simulink library "limbo_algorithm_atomic_sub_chart_library"  (R2013b)
settings: Solver=ode45  StartTime=0.0  StopTime=10.0  RelTol=1e-3
libraries: legonxtlib x1
settings Model: Creator=mbiesiad  LastModifiedBy=grouleau

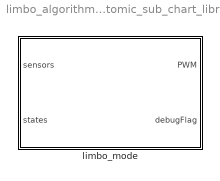
== system limbo_algorithm_atomic_sub_chart_library ==
  limbo_mode : Stateflow chart  TreatAsAtomicUnit=on

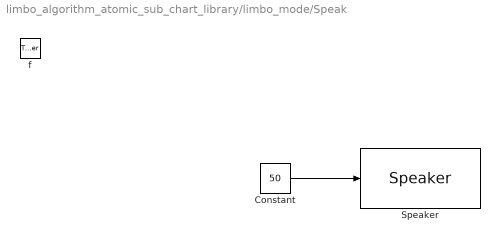
== system limbo_algorithm_atomic_sub_chart_library/limbo_mode/Speak ==
  f : TriggerPort  TriggerType=function-call
      settings: CopyFcn=Stateflow.SLINSF.SimulinkMan.removeBlockPreDeleteFcn  PreDeleteFcn=Stateflow.SLINSF.SimulinkMan.unsafePredeleteFcn
  Constant : Constant  Value=50
  Speaker : legonxtlib/Speaker  sinputMode=Volume only  sspeakerFreq=800  sspeakerVolume=50  sspeakerDuration=100
  wires:
  Constant/1 -> Speaker/1

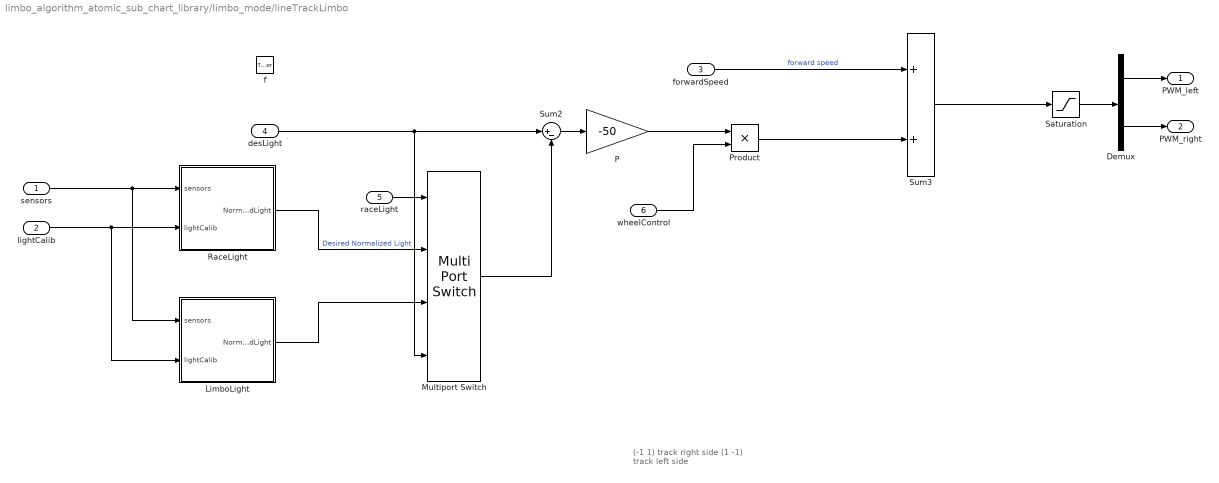
== system limbo_algorithm_atomic_sub_chart_library/limbo_mode/lineTrackLimbo ==
  note: (-1 1)  track right side
      | (1 -1)  track left side
  sensors : Inport  OutDataTypeStr=Bus: Sensors_Bus  PortDimensions=1  LockScale=on
  lightCalib : Inport  Port=2  OutDataTypeStr=Bus: Light_Bus  PortDimensions=1
  forwardSpeed : Inport  Port=3  OutDataTypeStr=single  PortDimensions=[1 2]
  desLight : Inport  Port=4  OutDataTypeStr=single  PortDimensions=1
  raceLight : Inport  Port=5  OutDataTypeStr=single  PortDimensions=1
  wheelControl : Inport  Port=6  OutDataTypeStr=single  PortDimensions=[1 2]
  f : TriggerPort  TriggerType=function-call
      settings: CopyFcn=Stateflow.SLINSF.SimulinkMan.removeBlockPreDeleteFcn  PreDeleteFcn=Stateflow.SLINSF.SimulinkMan.unsafePredeleteFcn
  Demux : Demux  Outputs=2
  LimboLight : Subsystem
  Multiport Switch : MultiPortSwitch
  P : Gain  Gain=-50
  Product : Product
  RaceLight : Subsystem
  Saturation : Saturate  UpperLimit=100  LowerLimit=-100  OutDataTypeStr=single
  Sum2 : Sum  Inputs=|+-
  Sum3 : Sum
  PWM_left : Outport  OutDataTypeStr=single  PortDimensions=1
  PWM_right : Outport  Port=2  OutDataTypeStr=single  PortDimensions=1
  wires:
  Saturation/1 -> Demux/1
  P/1 -> Product/1
  forwardSpeed/1 -> Sum3/1  "forward speed"
  Demux/2 -> PWM_right/1
  Demux/1 -> PWM_left/1
  Sum2/1 -> P/1
  desLight/1 -> Multiport Switch/4, Sum2/1  "Desired Normalized Light"
  sensors/1 -> LimboLight/1(sensors), RaceLight/1(sensors)
  lightCalib/1 -> LimboLight/2(lightCalib), RaceLight/2(lightCalib)
  LimboLight/1(NormalizedLight) -> Multiport Switch/3
  raceLight/1 -> Multiport Switch/1
  RaceLight/1(NormalizedLight) -> Multiport Switch/2
  Multiport Switch/1 -> Sum2/2
  wheelControl/1 -> Product/2
  Sum3/1 -> Saturation/1
  Product/1 -> Sum3/2

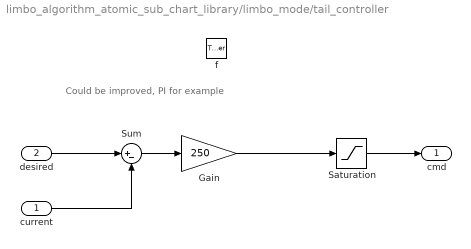
== system limbo_algorithm_atomic_sub_chart_library/limbo_mode/tail_controller ==
  note: Could be improved, PI for example
  current : Inport  OutDataTypeStr=single  PortDimensions=1
  desired : Inport  Port=2  OutDataTypeStr=single  PortDimensions=1
  f : TriggerPort  TriggerType=function-call
      settings: CopyFcn=Stateflow.SLINSF.SimulinkMan.removeBlockPreDeleteFcn  PreDeleteFcn=Stateflow.SLINSF.SimulinkMan.unsafePredeleteFcn
  Gain : Gain  Gain=250
  Saturation : Saturate  UpperLimit=100  LowerLimit=-100  OutDataTypeStr=single
  Sum : Sum  Inputs=|+-
  cmd : Outport  OutDataTypeStr=single  PortDimensions=1  InitialOutput=0
  wires:
  Sum/1 -> Gain/1
  current/1 -> Sum/2
  desired/1 -> Sum/1
  Gain/1 -> Saturation/1
  Saturation/1 -> cmd/1

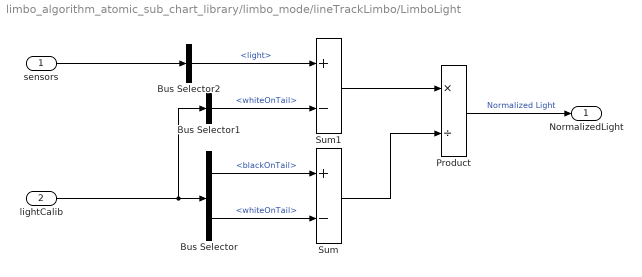
== system limbo_algorithm_atomic_sub_chart_library/limbo_mode/lineTrackLimbo/LimboLight ==
  sensors : Inport  OutDataTypeStr=Bus: Sensors_Bus  PortDimensions=1  LockScale=on
  lightCalib : Inport  Port=2  OutDataTypeStr=Bus: Light_Bus  PortDimensions=1
  Bus Selector : BusSelector  OutputSignals=blackOnTail,whiteOnTail
  Bus Selector1 : BusSelector  OutputSignals=whiteOnTail
  Bus Selector2 : BusSelector  OutputSignals=light
  Product : Product  Inputs=*/
  Sum : Sum  Inputs=+-
  Sum1 : Sum  Inputs=+-
  NormalizedLight : Outport
  wires:
  Product/1 -> NormalizedLight/1  "Normalized Light"
  Bus Selector2/1 -> Sum1/1  "<light>"
  sensors/1 -> Bus Selector2/1
  lightCalib/1 -> Bus Selector1/1, Bus Selector/1
  Bus Selector/2 -> Sum/2  "<whiteOnTail>"
  Bus Selector/1 -> Sum/1  "<blackOnTail>"
  Sum/1 -> Product/2
  Bus Selector1/1 -> Sum1/2  "<whiteOnTail>"
  Sum1/1 -> Product/1

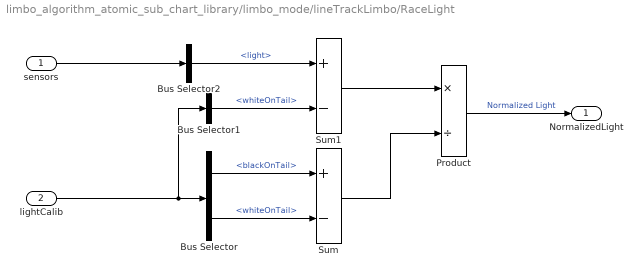
== system limbo_algorithm_atomic_sub_chart_library/limbo_mode/lineTrackLimbo/RaceLight ==
  sensors : Inport  OutDataTypeStr=Bus: Sensors_Bus  PortDimensions=1  LockScale=on
  lightCalib : Inport  Port=2  OutDataTypeStr=Bus: Light_Bus  PortDimensions=1
  Bus Selector : BusSelector  OutputSignals=blackOnTail,whiteOnTail
  Bus Selector1 : BusSelector  OutputSignals=whiteOnTail
  Bus Selector2 : BusSelector  OutputSignals=light
  Product : Product  Inputs=*/
  Sum : Sum  Inputs=+-
  Sum1 : Sum  Inputs=+-
  NormalizedLight : Outport
  wires:
  Sum1/1 -> Product/1
  Bus Selector1/1 -> Sum1/2  "<whiteOnTail>"
  Sum/1 -> Product/2
  Bus Selector/1 -> Sum/1  "<blackOnTail>"
  Bus Selector/2 -> Sum/2  "<whiteOnTail>"
  lightCalib/1 -> Bus Selector/1, Bus Selector1/1
  sensors/1 -> Bus Selector2/1
  Bus Selector2/1 -> Sum1/1  "<light>"
  Product/1 -> NormalizedLight/1  "Normalized Light"

== stateflow chart limbo_algorithm_atomic_sub_chart_library/limbo_mode ==
  state limbo_mode
    entry:
    desired_tail = single(1.6);
    raceLight = single(1);
    wheelControl = single([-1 1]);
    entry, during, exit:
    PWM.tail = tail_controller(sensors.theta_T, desired_tail);
    [PWM.left, PWM.right] = lineTrackLimbo(sensors, lightCalib, speed_ref, desLight, raceLight, wheelControl);
    state Approach
      entry:
      debugFlag = uint16(1100);
      Speak;
      speed_ref = single([25 25]);
      desLight = single(0.25);
    state TiltDown
      entry:
      debugFlag = uint16(1101);
      Speak;
      speed_ref = single([0 0]);
      during:
      desired_tail = desired_tail - single(0.3/(2/0.004));
    state FirstGate
      entry:
      debugFlag = uint16(1102);
      Speak;
      raceLight = single(2);
      desLight = single(0.5);
      speed_ref = single([20 20]);
    state TiltUpMoon1
      entry:
      debugFlag = uint16(1102);
      speed_ref = single([0 0]);
      desired_tail = single(1.7);
    state FirstHalfMoon
      entry:
      debugFlag = uint16(1103);
      Speak;
      raceLight = single(3);
      speed_ref = single([45 -30]);
      phi_save = states.phi;
    state SecondGateApproach
      entry:
      debugFlag = uint16(1100);
      raceLight = single(1);
      speed_ref = single([15 15]);
      desLight = single(0.5);
    state SecondGate
      entry:
      debugFlag = uint16(1103);
      Speak;
      raceLight = single(2);
      speed_ref = single([20 20]);
    state TiltDownMoon1
      entry:
      debugFlag = uint16(1101);
      speed_ref = single([0 0]);
      during:
      desired_tail = desired_tail - single(0.3/(2/0.004));
    state TiltUpMoon2
      entry:
      debugFlag = uint16(1102);
      speed_ref = single([0 0]);
      desired_tail = single(1.7);
    state SecondHalfMoon
      entry:
      debugFlag = uint16(1103);
      Speak;
      raceLight = single(3);
      speed_ref = single([45 -30]);
      phi_save = states.phi;
    state ThirdGateApproach
      entry:
      debugFlag = uint16(1100);
      raceLight = single(1);
      speed_ref = single([15 15]);
      desLight = single(0.3);
    state ThirdGate
      entry:
      debugFlag = uint16(1103);
      Speak;
      desLight = single(0.5);
      raceLight = single(2);
      speed_ref = single([20 20]);
    state TiltDownMoon2
      entry:
      debugFlag = uint16(1101);
      speed_ref = single([0 0]);
      during:
      desired_tail = desired_tail - single(0.3/(2/0.004));
    state TiltUp
      entry:
      debugFlag = uint16(1103);
      Speak;
      speed_ref = single([0 0]);
      desired_tail = single(1.6);
      %during:
      %desired_tail = desired_tail + single(0.3/(1/0.004));
    state Kick
      entry:
      debugFlag = uint16(1104);
      Speak;
      raceLight = single(1);
      speed_ref = single([45 45]);
      desLight = single(0.3);
      saveTheta = states.balancerStates.theta;
      during:
      debugFlag = uint16(abs(states.balancerStates.theta - saveTheta));
    state LimboDone1
      entry:
      debugFlag = uint16(1105);
      Speak;
      speed_ref = single([0 0]);
    state LimboDone
      entry:
      debugFlag = uint16(1105);
      Speak;
      speed_ref = single([0 0]);
      current_mode_status =OperationModeStatusEnum.SUCCESSFULLY_COMPLETED;
    (default) -> Approach
    Approach -> TiltDown : [sensors.sonar < single(10)]
    TiltDown -> FirstGate : [desired_tail <= 1.1]
    FirstGate -> TiltUpMoon1 : after(3, sec)
    TiltUpMoon1 -> FirstHalfMoon : after(0.5, sec)
    FirstHalfMoon -> SecondGateApproach : [abs(states.phi - phi_save) >= pi]
    SecondGateApproach -> TiltDownMoon1 : [sensors.sonar < single(10)]
    TiltDownMoon1 -> SecondGate : [desired_tail <= 1.1]
    SecondGate -> TiltUpMoon2 : after(4, sec)
    TiltUpMoon2 -> SecondHalfMoon : after(0.5, sec)
    SecondHalfMoon -> ThirdGateApproach : [abs(states.phi - phi_save) >= pi]
    ThirdGateApproach -> TiltDownMoon2 : [sensors.sonar < single(10)]
    TiltDownMoon2 -> ThirdGate : [desired_tail <= 1.1]
    ThirdGate -> TiltUp : after(4, sec)
    TiltUp -> Kick : after(0.5, sec)
    Kick -> LimboDone1 : [abs(states.balancerStates.theta - saveTheta) > single(47)]
  state cmd = tail_controller(current,desired) [function]
  state [PWM_left,PWM_right] = lineTrackLimbo(sensors,lightCalib,forwardSpeed,desLight,raceLight,wheelControl) [function]
  state Speak [function]
  data: current function_input single size=1; desired function_input single size=1; cmd function_output single size=1; sensors function_input Bus: Sensors_Bus size=1; lightCalib function_input Bus: Light_Bus size=1; PWM_left function_output single size=1; PWM_right function_output single size=1; forwardSpeed function_input single size=[1 2]; desLight function_input single size=1; raceLight function_input single size=1; wheelControl function_input single size=[1 2]; sensors input Bus: Sensors_Bus size=1; lightCalib data_store_memory; PWM output Bus: PWM_bus size=1; debugFlag output uint16 size=1; current_mode_status data_store_memory; desLight local size=1; speed_ref local size=[1 2]; desired_tail local size=1; raceLight local; states input Bus: States_Bus; wheelControl local; phi_save local; saveTheta local
